simulink model "ModeAdjust"  (R2018b)
settings: Solver=FixedStepDiscrete  StartTime=0.0  StopTime=inf  FixedStep=0.01  RelTol=1e-3
undefined symbols (not defined in the file or in its folder): IfKeSMSbSeatMovBkRclnEnable_Val, IfKeSMSbSeatMovFrwdBkwdEnable_Val, IfKeSMSbSeatMovFtrstEnable_Val, IfKeSMSbSeatMovHdrstFrwdBkwdEnable_Val, IfKeSMSbSeatMovHdUpwdDnwdEnable_Val, IfKeSMSbSeatMovLgrstEnable_Val, IfKeSMSbSeatMovLtwdRtwdEnable_Val, IfVeSMSeStNumConfig, KeSMSbArmscreenMovEnable_Val, KeSMSbSeatMovLgrstExpdEnable_Val, KeSMSuFirstRwStBackPosDelta_Val, KeSMSuFirstRwStBackPosTolr_Val, KeSMSuFirstRwStCushFrntPosDelta_Val, KeSMSuFirstRwStCushFrntPosTolr_Val, KeSMSuFirstRwStCushRePosDelta_Val, KeSMSuFirstRwStCushRePosTolr_Val, KeSMSuFirstRwStFootrestPosDelta_Val, KeSMSuFirstRwStFootrestPosTolr_Val, KeSMSuFirstRwStFwdBkwdPosDelta_Val, KeSMSuFirstRwStFwdBkwdPosTolr_Val, KeSMSuMdMotFinshdTm_Val, KeSMSuMdRetryTm1_Val, KeSMSuModeReqDurgTm_Val, KeSMSuSecRwStArmTochPosDelta_Val, KeSMSuSecRwStArmTochPosTolr_Val, KeSMSuSecRwStBackPosDelta_Val, KeSMSuSecRwStBackPosTolr_Val, KeSMSuSecRwStFtrstUpwdDnwdPosDelta_Val, KeSMSuSecRwStFtrstUpwdDnwdPosTolr_Val, KeSMSuSecRwStFwdBkwdPosDelta_Val, KeSMSuSecRwStFwdBkwdPosTolr_Val, KeSMSuSecRwStHeadrestFwdBkwdPosDelta_Val, KeSMSuSecRwStHeadrestFwdBkwdPosTolr_Val, KeSMSuSecRwStHeadrestUpwdDwnwdPosDelta_Val, KeSMSuSecRwStHeadrestUpwdDwnwdPosTolr_Val, KeSMSuSecRwStLegrestInOutPosDelta_Val, KeSMSuSecRwStLegrestInOutPosTolr_Val, KeSMSuSecRwStLegrestUpwdDwnwdPosDelta_Val, KeSMSuSecRwStLegrestUpwdDwnwdPosTolr_Val, KeSMSuSecRwStLwdRwdPosDelta_Val, KeSMSuSecRwStLwdRwdPosTolr_Val, KeSMSuSecRwStVIPFtrstRefAngle_Val, KeSMSuThirdRwStFwdBkwdPosDelta_Val, KeSMSuThirdRwStFwdBkwdPosTolr_Val, KeSMSuThrdRwCushFoldPosDelta_Val, KeSMSuThrdRwCushFoldPosTolr_Val, KeSMSuThrdRwStBackPosDelta_Val, KeSMSuThrdRwStBackPosTolr_Val, KeSMSw4SLegrstCloseMdSecRwLtStFtrstUpwdDnwdPos_Val, KeSMSw4SLegrstCloseMdSecRwLtStFtrstUpwdDnwdPosMax_Val, KeSMSw4SLegrstCloseMdSecRwLtStFtrstUpwdDnwdPosMin_Val, KeSMSw4SLegrstCloseMdSecRwLtStLgrstOtwdInwdPos_Val, KeSMSw4SLegrstCloseMdSecRwLtStLgrstOtwdInwdPosMax_Val, KeSMSw4SLegrstCloseMdSecRwLtStLgrstOtwdInwdPosMin_Val, KeSMSw4SLegrstCloseMdSecRwLtStLgrstUpwdDnwdPos_Val, KeSMSw4SLegrstCloseMdSecRwLtStLgrstUpwdDnwdPosMax_Val, KeSMSw4SLegrstCloseMdSecRwLtStLgrstUpwdDnwdPosMin_Val, KeSMSw4SLegrstCloseMdSecRwRtStFtrstUpwdDnwdPos_Val, KeSMSw4SLegrstCloseMdSecRwRtStFtrstUpwdDnwdPosMax_Val, KeSMSw4SLegrstCloseMdSecRwRtStFtrstUpwdDnwdPosMin_Val ... (+1138)
libraries: Lib x401
(part 18 of 35)

== system ModeAdjust/ModeAdjustRunnable_sys/ModeAdjust/LgrstOpenL/R2Lt ==
  note: 2L 扶手屏位置
  Mode_Trig : Inport
  SecRwLtStsPoss : Inport  Port=2
  SecRwLtStPossV : Inport  Port=3
  ModeStCalib_2L : Inport  Port=4
  StConfig : Inport  Port=5
  SecRwLtStsPoss4s : Inport  Port=6
  SecRwLtStPossV4s : Inport  Port=7
  StConfig4s : Inport  Port=8
  StepEn_LgrstStep1 : Inport  Port=9
  StepEn_LgrstStep2 : Inport  Port=10
  StepEn_LgrstStep3 : Inport  Port=11
  Bus Creator : BusCreator  Inputs=9  OutDataTypeStr=Bus: SecRwLfSeatPos
  Bus Creator1 : BusCreator  Inputs=3
  Bus Selector : BusSelector  OutputSignals=IfVeSMSuSecRwLtStBkReclnUpwdDnwdPos_Val_read,IfVeSMSuSecRwLtStFrwdBkwdPos_Val_read,IfVeSMSuSecRwLtStHPassStUpwdDnwdPos_Val_read,IfVeSMSuSecRwLtStLgrstUpwdDnwdPos_Val_read,IfVeSMSuSecRwLtStLtwdRtwdPos_Val_read,IfVeSMSuSecRwLtStArmScrnPos_Val_read
  Bus Selector1 : BusSelector  OutputSignals=IfVeSMSuSecRwLtStBkReclnUpwdDnwdPosV_Val_read,IfVeSMSuSecRwLtStFrwdBkwdPosV_Val_read,IfVeSMSuSecRwLtStHPassStUpwdDnwdPosV_Val_read,IfVeSMSuSecRwLtStLgrstUpwdDnwdPosV_Val_read,IfVeSMSuSecRwLtStLtwdRtwdPosV_Val_read,IfVeSMSuSecRwLtStArmScrnPosV_Val_read
  Bus Selector2 : BusSelector  OutputSignals=BkReclnUpwdDnwdPos,BkReclnUpwdDnwdPosMax,BkReclnUpwdDnwdPosMin,HdrstUpwdPos,HdrstUpwdPosMax,HdrstUpwdPosMin,LgrstUpwdPos,LgrstUpwdPosMax,LgrstUpwdPosMin,LgrstOtwdInwdPos,LgrstOtwdInwdPosMax,LgrstOtwdInwdPosMin,FtrstUpwdDnwdPos,FtrstUpwdDnwdPosMax,FtrstUpwdDnwdPosMin,HdrstFrwdBkwdnwdPos,HdrstFrwdBkwdnwdPosMax,HdrstFrwdBkwdnwdPosMin
  Bus Selector3 : BusSelector  OutputSignals=LgrstOpenLSecRwLtSt
  Bus Selector4 : BusSelector  OutputSignals=BkReclnUpwdDnwdMovConfig,ArmTouchMovConfig,FrwdBkwdMovConfig,LgrstUpwdMovConfig,LtwdRtwdMovConfig
  Bus Selector5 : BusSelector  OutputSignals=IfVeSMSuSecRwLtStLgrstOtwdInwdPos_Val_read,IfVeSMSuRrLtStFtUpwdDnwdPos_Val_read,IfVeSMSuSecRwLtStHdrstFrwdBkwdPos_Val_read
  Bus Selector6 : BusSelector  OutputSignals=IfVeSMSuSecRwLtStLgrstOtwdInwdPosV_Val_read,IfVeSMSuRrLtStFtUpwdDnwdPosV_Val_read,IfVeSMSuSecRwLtStHdrstFrwdBkwdPosV_Val_read
  Bus Selector7 : BusSelector  OutputSignals=LgrstExpdMovConfig,FtrstMovConfig,HdrstUpwdDnwdMovConfig,HdrstFrwdBkwdMovConfig
  Logical Operator10 : Logic  AllPortsSameDT=off  OutDataTypeStr=boolean
  Logical Operator4 : Logic  Operator=OR  AllPortsSameDT=off  OutDataTypeStr=boolean
  Logical Operator5 : Logic  Operator=OR  AllPortsSameDT=off  OutDataTypeStr=boolean
  Logical Operator6 : Logic  Operator=OR  AllPortsSameDT=off  OutDataTypeStr=boolean
  PA_KeSMSuMdMotFinshdTm_Val : Constant  Value=KeSMSuMdMotFinshdTm_Val
  PA_KeSMSuMdRetryTm1_Val : Constant  Value=KeSMSuMdRetryTm1_Val
  PA_KeSMSuModeReqDurgTm_Val : Constant  Value=KeSMSuModeReqDurgTm_Val
  PA_KeSMSuSecRwStBackPosDelta_Val : Constant  Value=KeSMSuSecRwStBackPosDelta_Val
  PA_KeSMSuSecRwStFtrstUpwdDnwdPosDelta_Val : Constant  Value=KeSMSuSecRwStFtrstUpwdDnwdPosDelta_Val
  PA_KeSMSuSecRwStHeadrestFwdBkwdPosDelta_Val : Constant  Value=KeSMSuSecRwStHeadrestFwdBkwdPosDelta_Val
  PA_KeSMSuSecRwStHeadrestUpwdDwnwdPosDelta_Val : Constant  Value=KeSMSuSecRwStHeadrestUpwdDwnwdPosDelta_Val
  PA_KeSMSuSecRwStLegrestInOutPosDelta_Val : Constant  Value=KeSMSuSecRwStLegrestInOutPosDelta_Val
  PA_KeSMSuSecRwStLegrestUpwdDwnwdPosDelta_Val : Constant  Value=KeSMSuSecRwStLegrestUpwdDwnwdPosDelta_Val
  PA_KeSMSwDltTrgtPos_Val{1,3,5..8,12..13,16,18..20} (12 alike) : Constant  Value=KeSMSwPosInvalidVal_Val
  PA_KeSMSwDltTrgtPos_Val{9..11,14..15,22} (6 alike) : Constant  Value=0  OutDataTypeStr=boolean
  PA_KeSMSwDltTrgtPos_Val4 : Constant  OutDataTypeStr=boolean
  SecRwLtStFtUpwd_Lt_Step2 : Lib/CommonUsed  SystemSampleTime=-1
  SecRwLtStLgrstOtwd_Lt_Step1 : Lib/CommonUsed  SystemSampleTime=-1
  SecRwLtStLgrstUpwd_Lt_Step3 : Lib/CommonUsed  SystemSampleTime=-1
  Unit Delay : UnitDelay  SampleTime=-1
  Unit Delay1 : UnitDelay  SampleTime=-1
  Unit Delay2 : UnitDelay  SampleTime=-1
  R2Lt_TrgtPoss : Outport  VectorParamsAs1DForOutWhenUnconnected=on
  IfVeSMSuSecRwLtStRclCmdSrv_Val_writeRaw : Outport  Port=2
  lgrstStep1_ini : Outport  Port=3  VectorParamsAs1DForOutWhenUnconnected=on
  lgrstStep2_ini : Outport  Port=4  VectorParamsAs1DForOutWhenUnconnected=on
  lgrstStep3_ini : Outport  Port=5  VectorParamsAs1DForOutWhenUnconnected=on
  lgrstStep1_done : Outport  Port=6  VectorParamsAs1DForOutWhenUnconnected=on
  lgrstStep2_done : Outport  Port=7  VectorParamsAs1DForOutWhenUnconnected=on
  lgrstStep3_done : Outport  Port=8  VectorParamsAs1DForOutWhenUnconnected=on
  R2Lt_TrgtPoss_2 : Outport  Port=9  VectorParamsAs1DForOutWhenUnconnected=on
  wires:
  PA_KeSMSuSecRwStHeadrestFwdBkwdPosDelta_Val/1 -> [KeSMSuSecRwStHeadrestFwdBkwdPosDelta_Val]
  Bus Selector2/18 -> [K_HdrstFrwdBkwdnwdPosMin]  "<HdrstFrwdBkwdnwdPosMin>"
  Bus Selector2/17 -> [K_HdrstFrwdBkwdnwdPosMax]  "<HdrstFrwdBkwdnwdPosMax>"
  Bus Selector2/16 -> [K_HdrstFrwdBkwdnwdPos]  "<HdrstFrwdBkwdnwdPos>"
  Bus Selector6/3 -> [SecRwLtStHdrstFrwdBkwdPosV]  "<IfVeSMSuSecRwLtStHdrstFrwdBkwdPosV_Val_read>"
  Bus Selector5/3 -> [SecRwLtStHdrstFrwdBkwdPos]  "<IfVeSMSuSecRwLtStHdrstFrwdBkwdPos_Val_read>"
  Bus Selector7/4 -> [HdrstFrwdBkwdMovConfig]  "<HdrstFrwdBkwdMovConfig>"
  PA_KeSMSwDltTrgtPos_Val6/1 -> Bus Creator1/3  "SecRwLtStHdrstFrwdBkwdTrgtPos"
  PA_KeSMSuMdRetryTm1_Val/1 -> [CntLow]
  [CntLow] -> SecRwLtStLgrstUpwd_Lt_Step3/15
  [CntLow] -> SecRwLtStLgrstOtwd_Lt_Step1/15
  [CntLow] -> SecRwLtStFtUpwd_Lt_Step2/15
  PA_KeSMSwDltTrgtPos_Val4/1 -> IfVeSMSuSecRwLtStRclCmdSrv_Val_writeRaw/1
  SecRwLtStLgrstUpwd_Lt_Step3/1 -> [lgrstStep1_ini]
  Mode_Trig/1 -> [Trig]
  Bus Selector1/3 -> [SecRwLtStHPassStUpwdDnwdPosV]  "<IfVeSMSuSecRwLtStHPassStUpwdDnwdPosV_Val_read>"
  Bus Selector/5 -> [SecRwLtStLtwdRtwdPos]  "<IfVeSMSuSecRwLtStLtwdRtwdPos_Val_read>"
  SecRwLtStsPoss/1 -> Bus Selector/1
  Bus Selector1/4 -> [SecRwLtStLgrstUpwdDnwdPosV]  "<IfVeSMSuSecRwLtStLgrstUpwdDnwdPosV_Val_read>"
  SecRwLtStPossV/1 -> Bus Selector1/1
  Bus Selector/3 -> [SecRwLtStHPassStUpwdDnwdPos]  "<IfVeSMSuSecRwLtStHPassStUpwdDnwdPos_Val_read>"
  Bus Selector1/5 -> [SecRwLtStLtwdRtwdPosV]  "<IfVeSMSuSecRwLtStLtwdRtwdPosV_Val_read>"
  Bus Selector/4 -> [SecRwLtStLgrstUpwdDnwdPos]  "<IfVeSMSuSecRwLtStLgrstUpwdDnwdPos_Val_read>"
  Bus Selector/2 -> [SecRwLtStFrwdBkwdPos]  "<IfVeSMSuSecRwLtStFrwdBkwdPos_Val_read>"
  Bus Selector1/1 -> [SecRwLtStBkReclnUpwdDnwdPosV]  "<IfVeSMSuSecRwLtStBkReclnUpwdDnwdPosV_Val_read>"
  Bus Selector1/2 -> [SecRwLtStFrwdBkwdPosV]  "<IfVeSMSuSecRwLtStFrwdBkwdPosV_Val_read>"
  Bus Selector/1 -> [SecRwLtStBkReclnUpwdDnwdPos]  "<IfVeSMSuSecRwLtStBkReclnUpwdDnwdPos_Val_read>"
  [Trig] -> SecRwLtStLgrstUpwd_Lt_Step3/1
  [StepEn_LgrstStep1] -> SecRwLtStLgrstUpwd_Lt_Step3/2
  [K_LgrstUpwdPosMin] -> SecRwLtStLgrstUpwd_Lt_Step3/4
  [K_LgrstUpwdPosMax] -> SecRwLtStLgrstUpwd_Lt_Step3/5
  [K_LgrstUpwdPos] -> SecRwLtStLgrstUpwd_Lt_Step3/6
  [SecRwLtStLgrstUpwdDnwdPos] -> SecRwLtStLgrstUpwd_Lt_Step3/3
  [KeSMSuSecRwStLegrestUpwdDwnwdPosDelta_Val] -> SecRwLtStLgrstUpwd_Lt_Step3/7
  [SecRwLtStLgrstUpwdDnwdPosV] -> SecRwLtStLgrstUpwd_Lt_Step3/8
  PA_KeSMSwDltTrgtPos_Val10/1 -> SecRwLtStLgrstUpwd_Lt_Step3/9
  PA_KeSMSwDltTrgtPos_Val12/1 -> SecRwLtStLgrstUpwd_Lt_Step3/10
  [Tick] -> SecRwLtStLgrstUpwd_Lt_Step3/11
  SecRwLtStLgrstUpwd_Lt_Step3/2 -> [lgrst_ArrivedTarPos]
  SecRwLtStLgrstUpwd_Lt_Step3/3 -> [R2Lt_LgrstUpwd_TarPos]
  SecRwLtStLgrstUpwd_Lt_Step3/4 -> [lgrstStep1_done]
  PA_KeSMSwDltTrgtPos_Val3/1 -> Bus Creator/6  "SecRwLtStHdrstUpwdDnwdTrgtPos"
  Bus Creator/1 -> R2Lt_TrgtPoss/1
  [R2Lt_LgrstUpwd_TarPos] -> Bus Creator/7  "SecRwLtStLgrstUpwdDnwdTrgtPos"
  PA_KeSMSwDltTrgtPos_Val19/1 -> Bus Creator/3  "SecRwLtStCshnFrntUpwdDnwdTrgtPos"
  PA_KeSMSwDltTrgtPos_Val1/1 -> Bus Creator/8  "SecRwLtStLtwdRtwdTrgtPos"
  PA_KeSMSwDltTrgtPos_Val18/1 -> Bus Creator/2  "SecRwLtStBlstOtwdInwdTrgtPos"
  PA_KeSMSwDltTrgtPos_Val5/1 -> Bus Creator/1  "SecRwLtStBkReclnUpwdDnwdTrgtPos"
  PA_KeSMSwDltTrgtPos_Val8/1 -> Bus Creator/5  "SecRwLtStFrwdBkwdTrgtPos"
  PA_KeSMSwDltTrgtPos_Val20/1 -> Bus Creator/4  "SecRwLtStCshnRrUpwdDnwdTrgtPos"
  PA_KeSMSuModeReqDurgTm_Val/1 -> [Tick]
  PA_KeSMSwDltTrgtPos_Val7/1 -> Bus Creator/9  "SecRwLtStArmScrnTrgtPos"
  PA_KeSMSuSecRwStBackPosDelta_Val/1 -> [KeSMSuSecRwStBackPosDelta_Val]
  PA_KeSMSuSecRwStLegrestUpwdDwnwdPosDelta_Val/1 -> [KeSMSuSecRwStLegrestUpwdDwnwdPosDelta_Val]
  PA_KeSMSuMdMotFinshdTm_Val/1 -> [KeSMSuMdMotFinshdTm_Val]
  [KeSMSuMdMotFinshdTm_Val] -> SecRwLtStLgrstUpwd_Lt_Step3/12
  Bus Selector/6 -> [R2LtStArmScrnPos]  "<IfVeSMSuSecRwLtStArmScrnPos_Val_read>"
  Bus Selector1/6 -> [R2LtStArmScrnPosV]  "<IfVeSMSuSecRwLtStArmScrnPosV_Val_read>"
  Bus Selector2/9 -> [K_LgrstUpwdPosMin]  "<LgrstUpwdPosMin>"
  Bus Selector2/6 -> [K_HdrstUpwdPosMin]  "<HdrstUpwdPosMin>"
  Bus Selector2/7 -> [K_LgrstUpwdPos]  "<LgrstUpwdPos>"
  Bus Selector2/5 -> [K_HdrstUpwdPosMax]  "<HdrstUpwdPosMax>"
  Bus Selector2/8 -> [K_LgrstUpwdPosMax]  "<LgrstUpwdPosMax>"
  Bus Selector2/4 -> [K_HdrstUpwdPos]  "<HdrstUpwdPos>"
  Bus Selector2/1 -> [K_BkReclnUpwdDnwdPos]  "<BkReclnUpwdDnwdPos>"
  Bus Selector2/2 -> [K_BkReclnUpwdDnwdPosMax]  "<BkReclnUpwdDnwdPosMax>"
  Bus Selector3/1 -> Bus Selector2/1  "<LgrstOpenLSecRwLtSt>"
  Bus Selector2/3 -> [K_BkReclnUpwdDnwdPosMin]  "<BkReclnUpwdDnwdPosMin>"
  ModeStCalib_2L/1 -> Bus Selector3/1
  StConfig/1 -> Bus Selector4/1
  Bus Selector4/3 -> [FrwdBkwdMovConfig]  "<FrwdBkwdMovConfig>"
  Bus Selector4/5 -> [LtwdRtwdMovConfig]  "<LtwdRtwdMovConfig>"
  Bus Selector4/4 -> [LgrstUpwdMovConfig]  "<LgrstUpwdMovConfig>"
  Bus Selector4/2 -> [ArmTouchMovConfig]  "<ArmTouchMovConfig>"
  Bus Selector4/1 -> [BkReclnUpwdDnwdMovConfig]  "<BkReclnUpwdDnwdMovConfig>"
  PA_KeSMSwDltTrgtPos_Val9/1 -> SecRwLtStLgrstUpwd_Lt_Step3/13
  [LgrstUpwdMovConfig] -> SecRwLtStLgrstUpwd_Lt_Step3/14
  Bus Selector2/10 -> [K_LgrstOtwdInwdPos]  "<LgrstOtwdInwdPos>"
  Bus Selector2/11 -> [K_LgrstOtwdInwdPosMax]  "<LgrstOtwdInwdPosMax>"
  Bus Selector2/12 -> [K_LgrstOtwdInwdPosMin]  "<LgrstOtwdInwdPosMin>"
  Bus Selector2/15 -> [K_FtrstUpwdPosMin]  "<FtrstUpwdDnwdPosMin>"
  Bus Selector2/14 -> [K_FtrstUpwdPosMax]  "<FtrstUpwdDnwdPosMax>"
  Bus Selector2/13 -> [K_FtrstUpwdPos]  "<FtrstUpwdDnwdPos>"
  PA_KeSMSuSecRwStFtrstUpwdDnwdPosDelta_Val/1 -> [KeSMSuSecRwStFtrstUpwdDnwdPosDelta_Val]
  PA_KeSMSuSecRwStHeadrestUpwdDwnwdPosDelta_Val/1 -> [KeSMSuSecRwStHeadrestUpwdDwnwdPosDelta_Val]
  PA_KeSMSuSecRwStLegrestInOutPosDelta_Val/1 -> [KeSMSuSecRwStLegrestInOutPosDelta_Val]
  SecRwLtStsPoss4s/1 -> Bus Selector5/1
  SecRwLtStPossV4s/1 -> Bus Selector6/1
  Bus Selector5/1 -> [SecRwLtStLgrstOtwdInwdPos]  "<IfVeSMSuSecRwLtStLgrstOtwdInwdPos_Val_read>"
  Bus Selector5/2 -> [RrLtStFtUpwdDnwdPos]  "<IfVeSMSuRrLtStFtUpwdDnwdPos_Val_read>"
  Bus Selector6/1 -> [SecRwLtStLgrstOtwdInwdPosV]  "<IfVeSMSuSecRwLtStLgrstOtwdInwdPosV_Val_read>"
  Bus Selector6/2 -> [RrLtStFtUpwdDnwdPosV]  "<IfVeSMSuRrLtStFtUpwdDnwdPosV_Val_read>"
  [LgrstExpdMovConfig] -> SecRwLtStLgrstOtwd_Lt_Step1/14
  PA_KeSMSwDltTrgtPos_Val15/1 -> SecRwLtStLgrstOtwd_Lt_Step1/13
  [KeSMSuMdMotFinshdTm_Val] -> SecRwLtStLgrstOtwd_Lt_Step1/12
  SecRwLtStLgrstOtwd_Lt_Step1/4 -> [LgrstStep3_1_done]
  SecRwLtStLgrstOtwd_Lt_Step1/3 -> [R2Lt_LgrstOtwd_TarPos]
  SecRwLtStLgrstOtwd_Lt_Step1/2 -> [LgOt_ArrivedTarPos]
  [Tick] -> SecRwLtStLgrstOtwd_Lt_Step1/11
  PA_KeSMSwDltTrgtPos_Val13/1 -> SecRwLtStLgrstOtwd_Lt_Step1/10
  PA_KeSMSwDltTrgtPos_Val14/1 -> SecRwLtStLgrstOtwd_Lt_Step1/9
  [SecRwLtStLgrstOtwdInwdPosV] -> SecRwLtStLgrstOtwd_Lt_Step1/8
  [KeSMSuSecRwStLegrestInOutPosDelta_Val] -> SecRwLtStLgrstOtwd_Lt_Step1/7
  [SecRwLtStLgrstOtwdInwdPos] -> SecRwLtStLgrstOtwd_Lt_Step1/3
  [K_LgrstOtwdInwdPos] -> SecRwLtStLgrstOtwd_Lt_Step1/6
  [K_LgrstOtwdInwdPosMax] -> SecRwLtStLgrstOtwd_Lt_Step1/5
  [K_LgrstOtwdInwdPosMin] -> SecRwLtStLgrstOtwd_Lt_Step1/4
  [StepEn_LgrstStep3] -> SecRwLtStLgrstOtwd_Lt_Step1/2
  [Trig] -> SecRwLtStLgrstOtwd_Lt_Step1/1
  SecRwLtStLgrstOtwd_Lt_Step1/1 -> [LgrstStep3_1_ini]
  SecRwLtStFtUpwd_Lt_Step2/1 -> [LgrstStep2_1_ini]
  [Trig] -> SecRwLtStFtUpwd_Lt_Step2/1
  [StepEn_LgrstStep2] -> SecRwLtStFtUpwd_Lt_Step2/2
  [K_FtrstUpwdPosMin] -> SecRwLtStFtUpwd_Lt_Step2/4
  [K_FtrstUpwdPosMax] -> SecRwLtStFtUpwd_Lt_Step2/5
  [K_FtrstUpwdPos] -> SecRwLtStFtUpwd_Lt_Step2/6
  [RrLtStFtUpwdDnwdPos] -> SecRwLtStFtUpwd_Lt_Step2/3
  [KeSMSuSecRwStFtrstUpwdDnwdPosDelta_Val] -> SecRwLtStFtUpwd_Lt_Step2/7
  [RrLtStFtUpwdDnwdPosV] -> SecRwLtStFtUpwd_Lt_Step2/8
  PA_KeSMSwDltTrgtPos_Val11/1 -> SecRwLtStFtUpwd_Lt_Step2/9
  PA_KeSMSwDltTrgtPos_Val16/1 -> SecRwLtStFtUpwd_Lt_Step2/10
  [Tick] -> SecRwLtStFtUpwd_Lt_Step2/11
  SecRwLtStFtUpwd_Lt_Step2/2 -> [Ft_ArrivedTarPos]
  SecRwLtStFtUpwd_Lt_Step2/3 -> [R2Lt_FtUpwd_TarPos]
  SecRwLtStFtUpwd_Lt_Step2/4 -> [LgrstStep2_1_done]
  [KeSMSuMdMotFinshdTm_Val] -> SecRwLtStFtUpwd_Lt_Step2/12
  PA_KeSMSwDltTrgtPos_Val22/1 -> SecRwLtStFtUpwd_Lt_Step2/13
  [FtrstMovConfig] -> SecRwLtStFtUpwd_Lt_Step2/14
  StConfig4s/1 -> Bus Selector7/1
  Bus Selector7/1 -> [LgrstExpdMovConfig]  "<LgrstExpdMovConfig>"
  Bus Selector7/2 -> [FtrstMovConfig]  "<FtrstMovConfig>"
  Bus Selector7/3 -> [HdrstMovConfig]  "<HdrstUpwdDnwdMovConfig>"
  [lgrstStep1_ini] -> lgrstStep1_ini/1
  [LgrstStep2_1_ini] -> lgrstStep2_ini/1
  [LgrstStep3_1_ini] -> lgrstStep3_ini/1
  StepEn_LgrstStep1/1 -> [StepEn_LgrstStep1]
  StepEn_LgrstStep2/1 -> [StepEn_LgrstStep2]
  StepEn_LgrstStep3/1 -> [StepEn_LgrstStep3]
  [LgrstStep2_1_done] -> Unit Delay1/1
  Logical Operator4/1 -> lgrstStep1_done/1
  [lgrstStep1_done] -> Unit Delay/1
  [lgrstStep1_ini] -> Logical Operator4/1
  Unit Delay/1 -> Logical Operator4/2
  Logical Operator5/1 -> [lgrst_Step2done], lgrstStep2_done/1
  Unit Delay1/1 -> Logical Operator5/2
  Logical Operator6/1 -> lgrstStep3_done/1
  Unit Delay2/1 -> Logical Operator6/2
  [LgrstStep3_1_done] -> Logical Operator10/2
  Logical Operator10/1 -> Unit Delay2/1
  [lgrst_Step2done] -> Logical Operator10/1
  [LgrstStep2_1_ini] -> Logical Operator5/1
  [LgrstStep3_1_ini] -> Logical Operator6/1
  Bus Creator1/1 -> R2Lt_TrgtPoss_2/1
  [R2Lt_FtUpwd_TarPos] -> Bus Creator1/1  "RrLtStFtUpwdDnwdTrgtPos"
  [R2Lt_LgrstOtwd_TarPos] -> Bus Creator1/2  "SecRwLtStLgrstOtwdInwdTrgtPos"

== system ModeAdjust/ModeAdjustRunnable_sys/ModeAdjust/LgrstOpenR/R2Lt ==
  note: 2L 扶手屏位置
  Mode_Trig : Inport
  SecRwLtStsPoss : Inport  Port=2
  SecRwLtStPossV : Inport  Port=3
  ModeStCalib_2L : Inport  Port=4
  StConfig : Inport  Port=5
  SecRwLtStsPoss4s : Inport  Port=6
  SecRwLtStPossV4s : Inport  Port=7
  StConfig4s : Inport  Port=8
  StepEn_LgrstStep1 : Inport  Port=9
  StepEn_LgrstStep2 : Inport  Port=10
  StepEn_LgrstStep3 : Inport  Port=11
  Bus Creator : BusCreator  Inputs=9  OutDataTypeStr=Bus: SecRwRtSeatPos
  Bus Creator1 : BusCreator  Inputs=3
  Bus Selector : BusSelector  OutputSignals=IfVeSMSuSecRwRtStBkReclnUpwdDnwdPos_Val_read,IfVeSMSuSecRwRtStFrwdBkwdPos_Val_read,IfVeSMSuSecRwRtStHPassStUpwdDnwdPos_Val_read,IfVeSMSuSecRwRtStLgrstUpwdDnwdPos_Val_read,IfVeSMSuSecRwRtStLtwdRtwdPos_Val_read,SecRwRtStArmScrnPos_Val_read
  Bus Selector1 : BusSelector  OutputSignals=IfVeSMSuSecRwRtStBkReclnUpwdDnwdPosV_Val_read,IfVeSMSuSecRwRtStFrwdBkwdPosV_Val_read,IfVeSMSuSecRwRtStHPassStUpwdDnwdPosV_Val_read,IfVeSMSuSecRwRtStLgrstUpwdDnwdPosV_Val_read,IfVeSMSuSecRwRtStLtwdRtwdPosV_Val_read,SecRwRtStArmScrnPosV_Val_read
  Bus Selector2 : BusSelector  OutputSignals=BkReclnUpwdDnwdPos,BkReclnUpwdDnwdPosMax,BkReclnUpwdDnwdPosMin,HdrstUpwdPos,HdrstUpwdPosMax,HdrstUpwdPosMin,LgrstUpwdPos,LgrstUpwdPosMax,LgrstUpwdPosMin,LgrstOtwdInwdPos,LgrstOtwdInwdPosMax,LgrstOtwdInwdPosMin,FtrstUpwdDnwdPos,FtrstUpwdDnwdPosMax,FtrstUpwdDnwdPosMin,HdrstFrwdBkwdnwdPos,HdrstFrwdBkwdnwdPosMax,HdrstFrwdBkwdnwdPosMin
  Bus Selector3 : BusSelector  OutputSignals=LgrstOpenRSecRwRtSt
  Bus Selector4 : BusSelector  OutputSignals=BkReclnUpwdDnwdMovConfig,ArmTouchMovConfig,FrwdBkwdMovConfig,LgrstUpwdMovConfig,LtwdRtwdMovConfig
  Bus Selector5 : BusSelector  OutputSignals=IfVeSMSuSecRwRtStLgrstOtwdInwdPos_Val_read,IfVeSMSuRrRtStFtUpwdDnwdPos_Val_read,IfVeSMSuSecRwRtStHdrstFrwdBkwdPos_Val_read
  Bus Selector6 : BusSelector  OutputSignals=IfVeSMSuSecRwRtStLgrstOtwdInwdPosV_Val_read,IfVeSMSuRrRtStFtUpwdDnwdPosV_Val_read,IfVeSMSuSecRwRtStHdrstFrwdBkwdPosV_Val_read
  Bus Selector7 : BusSelector  OutputSignals=LgrstExpdMovConfig,FtrstMovConfig,HdrstUpwdDnwdMovConfig,HdrstFrwdBkwdMovConfig
  Logical Operator10 : Logic  AllPortsSameDT=off  OutDataTypeStr=boolean
  Logical Operator4 : Logic  Operator=OR  AllPortsSameDT=off  OutDataTypeStr=boolean
  Logical Operator5 : Logic  Operator=OR  AllPortsSameDT=off  OutDataTypeStr=boolean
  Logical Operator6 : Logic  Operator=OR  AllPortsSameDT=off  OutDataTypeStr=boolean
  PA_KeSMSuMdMotFinshdTm_Val : Constant  Value=KeSMSuMdMotFinshdTm_Val
  PA_KeSMSuMdRetryTm1_Val : Constant  Value=KeSMSuMdRetryTm1_Val
  PA_KeSMSuModeReqDurgTm_Val : Constant  Value=KeSMSuModeReqDurgTm_Val
  PA_KeSMSuSecRwStBackPosDelta_Val : Constant  Value=KeSMSuSecRwStBackPosDelta_Val
  PA_KeSMSuSecRwStFtrstUpwdDnwdPosDelta_Val : Constant  Value=KeSMSuSecRwStFtrstUpwdDnwdPosDelta_Val
  PA_KeSMSuSecRwStHeadrestFwdBkwdPosDelta_Val : Constant  Value=KeSMSuSecRwStHeadrestFwdBkwdPosDelta_Val
  PA_KeSMSuSecRwStHeadrestUpwdDwnwdPosDelta_Val : Constant  Value=KeSMSuSecRwStHeadrestUpwdDwnwdPosDelta_Val
  PA_KeSMSuSecRwStLegrestInOutPosDelta_Val : Constant  Value=KeSMSuSecRwStLegrestInOutPosDelta_Val
  PA_KeSMSuSecRwStLegrestUpwdDwnwdPosDelta_Val : Constant  Value=KeSMSuSecRwStLegrestUpwdDwnwdPosDelta_Val
  PA_KeSMSwDltTrgtPos_Val{1,3,5..8,12..13,16,18..20} (12 alike) : Constant  Value=KeSMSwPosInvalidVal_Val
  PA_KeSMSwDltTrgtPos_Val{9..11,14..15,22} (6 alike) : Constant  Value=0  OutDataTypeStr=boolean
  PA_KeSMSwDltTrgtPos_Val4 : Constant  OutDataTypeStr=boolean
  SecRwLtStFtUpwd_Lt_Step2 : Lib/CommonUsed  SystemSampleTime=-1
  SecRwLtStLgrstOtwd_Lt_Step1 : Lib/CommonUsed  SystemSampleTime=-1
  SecRwLtStLgrstUpwd_Lt_Step3 : Lib/CommonUsed  SystemSampleTime=-1
  Unit Delay : UnitDelay  SampleTime=-1
  Unit Delay1 : UnitDelay  SampleTime=-1
  Unit Delay2 : UnitDelay  SampleTime=-1
  R2Rt_TrgtPoss : Outport  VectorParamsAs1DForOutWhenUnconnected=on
  IfVeSMSuSecRwLtStRclCmdSrv_Val_writeRaw : Outport  Port=2
  lgrstStep1_ini : Outport  Port=3  VectorParamsAs1DForOutWhenUnconnected=on
  lgrstStep2_ini : Outport  Port=4  VectorParamsAs1DForOutWhenUnconnected=on
  lgrstStep3_ini : Outport  Port=5  VectorParamsAs1DForOutWhenUnconnected=on
  lgrstStep1_done : Outport  Port=6  VectorParamsAs1DForOutWhenUnconnected=on
  lgrstStep2_done : Outport  Port=7  VectorParamsAs1DForOutWhenUnconnected=on
  lgrstStep3_done : Outport  Port=8  VectorParamsAs1DForOutWhenUnconnected=on
  R2Rt_TrgtPoss_2 : Outport  Port=9  VectorParamsAs1DForOutWhenUnconnected=on
  wires:
  [R2Lt_LgrstOtwd_TarPos] -> Bus Creator1/2  "SecRwRtStLgrstOtwdInwdTrgtPos"
  [R2Lt_FtUpwd_TarPos] -> Bus Creator1/1  "RrRtStFtUpwdDnwdTrgtPos"
  Bus Creator1/1 -> R2Rt_TrgtPoss_2/1
  [LgrstStep3_1_ini] -> Logical Operator6/1
  [LgrstStep2_1_ini] -> Logical Operator5/1
  [lgrst_Step2done] -> Logical Operator10/1
  Logical Operator10/1 -> Unit Delay2/1
  [LgrstStep3_1_done] -> Logical Operator10/2
  Unit Delay2/1 -> Logical Operator6/2
  Logical Operator6/1 -> lgrstStep3_done/1
  Unit Delay1/1 -> Logical Operator5/2
  Logical Operator5/1 -> lgrstStep2_done/1, [lgrst_Step2done]
  Unit Delay/1 -> Logical Operator4/2
  [lgrstStep1_ini] -> Logical Operator4/1
  [lgrstStep1_done] -> Unit Delay/1
  Logical Operator4/1 -> lgrstStep1_done/1
  [LgrstStep2_1_done] -> Unit Delay1/1
  StepEn_LgrstStep3/1 -> [StepEn_LgrstStep3]
  StepEn_LgrstStep2/1 -> [StepEn_LgrstStep2]
  StepEn_LgrstStep1/1 -> [StepEn_LgrstStep1]
  [LgrstStep3_1_ini] -> lgrstStep3_ini/1
  [LgrstStep2_1_ini] -> lgrstStep2_ini/1
  [lgrstStep1_ini] -> lgrstStep1_ini/1
  Bus Selector7/3 -> [HdrstMovConfig]  "<HdrstUpwdDnwdMovConfig>"
  Bus Selector7/2 -> [FtrstMovConfig]  "<FtrstMovConfig>"
  Bus Selector7/1 -> [LgrstExpdMovConfig]  "<LgrstExpdMovConfig>"
  StConfig4s/1 -> Bus Selector7/1
  [FtrstMovConfig] -> SecRwLtStFtUpwd_Lt_Step2/14
  PA_KeSMSwDltTrgtPos_Val22/1 -> SecRwLtStFtUpwd_Lt_Step2/13
  [KeSMSuMdMotFinshdTm_Val] -> SecRwLtStFtUpwd_Lt_Step2/12
  SecRwLtStFtUpwd_Lt_Step2/4 -> [LgrstStep2_1_done]
  SecRwLtStFtUpwd_Lt_Step2/3 -> [R2Lt_FtUpwd_TarPos]
  SecRwLtStFtUpwd_Lt_Step2/2 -> [Ft_ArrivedTarPos]
  [Tick] -> SecRwLtStFtUpwd_Lt_Step2/11
  PA_KeSMSwDltTrgtPos_Val16/1 -> SecRwLtStFtUpwd_Lt_Step2/10
  PA_KeSMSwDltTrgtPos_Val11/1 -> SecRwLtStFtUpwd_Lt_Step2/9
  [RrLtStFtUpwdDnwdPosV] -> SecRwLtStFtUpwd_Lt_Step2/8
  [KeSMSuSecRwStFtrstUpwdDnwdPosDelta_Val] -> SecRwLtStFtUpwd_Lt_Step2/7
  [RrLtStFtUpwdDnwdPos] -> SecRwLtStFtUpwd_Lt_Step2/3
  [K_FtrstUpwdPos] -> SecRwLtStFtUpwd_Lt_Step2/6
  [K_FtrstUpwdPosMax] -> SecRwLtStFtUpwd_Lt_Step2/5
  [K_FtrstUpwdPosMin] -> SecRwLtStFtUpwd_Lt_Step2/4
  [StepEn_LgrstStep2] -> SecRwLtStFtUpwd_Lt_Step2/2
  [Trig] -> SecRwLtStFtUpwd_Lt_Step2/1
  SecRwLtStFtUpwd_Lt_Step2/1 -> [LgrstStep2_1_ini]
  SecRwLtStLgrstOtwd_Lt_Step1/1 -> [LgrstStep3_1_ini]
  [Trig] -> SecRwLtStLgrstOtwd_Lt_Step1/1
  [StepEn_LgrstStep3] -> SecRwLtStLgrstOtwd_Lt_Step1/2
  [K_LgrstOtwdInwdPosMin] -> SecRwLtStLgrstOtwd_Lt_Step1/4
  [K_LgrstOtwdInwdPosMax] -> SecRwLtStLgrstOtwd_Lt_Step1/5
  [K_LgrstOtwdInwdPos] -> SecRwLtStLgrstOtwd_Lt_Step1/6
  [SecRwLtStLgrstOtwdInwdPos] -> SecRwLtStLgrstOtwd_Lt_Step1/3
  [KeSMSuSecRwStLegrestInOutPosDelta_Val] -> SecRwLtStLgrstOtwd_Lt_Step1/7
  [SecRwLtStLgrstOtwdInwdPosV] -> SecRwLtStLgrstOtwd_Lt_Step1/8
  PA_KeSMSwDltTrgtPos_Val14/1 -> SecRwLtStLgrstOtwd_Lt_Step1/9
  PA_KeSMSwDltTrgtPos_Val13/1 -> SecRwLtStLgrstOtwd_Lt_Step1/10
  [Tick] -> SecRwLtStLgrstOtwd_Lt_Step1/11
  SecRwLtStLgrstOtwd_Lt_Step1/2 -> [LgOt_ArrivedTarPos]
  SecRwLtStLgrstOtwd_Lt_Step1/3 -> [R2Lt_LgrstOtwd_TarPos]
  SecRwLtStLgrstOtwd_Lt_Step1/4 -> [LgrstStep3_1_done]
  [KeSMSuMdMotFinshdTm_Val] -> SecRwLtStLgrstOtwd_Lt_Step1/12
  PA_KeSMSwDltTrgtPos_Val15/1 -> SecRwLtStLgrstOtwd_Lt_Step1/13
  [LgrstExpdMovConfig] -> SecRwLtStLgrstOtwd_Lt_Step1/14
  Bus Selector6/2 -> [RrLtStFtUpwdDnwdPosV]  "<IfVeSMSuRrRtStFtUpwdDnwdPosV_Val_read>"
  Bus Selector6/1 -> [SecRwLtStLgrstOtwdInwdPosV]  "<IfVeSMSuSecRwRtStLgrstOtwdInwdPosV_Val_read>"
  Bus Selector5/2 -> [RrLtStFtUpwdDnwdPos]  "<IfVeSMSuRrRtStFtUpwdDnwdPos_Val_read>"
  Bus Selector5/1 -> [SecRwLtStLgrstOtwdInwdPos]  "<IfVeSMSuSecRwRtStLgrstOtwdInwdPos_Val_read>"
  SecRwLtStPossV4s/1 -> Bus Selector6/1
  SecRwLtStsPoss4s/1 -> Bus Selector5/1
  PA_KeSMSuSecRwStLegrestInOutPosDelta_Val/1 -> [KeSMSuSecRwStLegrestInOutPosDelta_Val]
  PA_KeSMSuSecRwStHeadrestUpwdDwnwdPosDelta_Val/1 -> [KeSMSuSecRwStHeadrestUpwdDwnwdPosDelta_Val]
  PA_KeSMSuSecRwStFtrstUpwdDnwdPosDelta_Val/1 -> [KeSMSuSecRwStFtrstUpwdDnwdPosDelta_Val]
  Bus Selector2/13 -> [K_FtrstUpwdPos]  "<FtrstUpwdDnwdPos>"
  Bus Selector2/14 -> [K_FtrstUpwdPosMax]  "<FtrstUpwdDnwdPosMax>"
  Bus Selector2/15 -> [K_FtrstUpwdPosMin]  "<FtrstUpwdDnwdPosMin>"
  Bus Selector2/12 -> [K_LgrstOtwdInwdPosMin]  "<LgrstOtwdInwdPosMin>"
  Bus Selector2/11 -> [K_LgrstOtwdInwdPosMax]  "<LgrstOtwdInwdPosMax>"
  Bus Selector2/10 -> [K_LgrstOtwdInwdPos]  "<LgrstOtwdInwdPos>"
  [LgrstUpwdMovConfig] -> SecRwLtStLgrstUpwd_Lt_Step3/14
  PA_KeSMSwDltTrgtPos_Val9/1 -> SecRwLtStLgrstUpwd_Lt_Step3/13
  Bus Selector4/1 -> [BkReclnUpwdDnwdMovConfig]  "<BkReclnUpwdDnwdMovConfig>"
  Bus Selector4/2 -> [ArmTouchMovConfig]  "<ArmTouchMovConfig>"
  Bus Selector4/4 -> [LgrstUpwdMovConfig]  "<LgrstUpwdMovConfig>"
  Bus Selector4/5 -> [LtwdRtwdMovConfig]  "<LtwdRtwdMovConfig>"
  Bus Selector4/3 -> [FrwdBkwdMovConfig]  "<FrwdBkwdMovConfig>"
  StConfig/1 -> Bus Selector4/1
  ModeStCalib_2L/1 -> Bus Selector3/1
  Bus Selector2/3 -> [K_BkReclnUpwdDnwdPosMin]  "<BkReclnUpwdDnwdPosMin>"
  Bus Selector3/1 -> Bus Selector2/1  "<LgrstOpenRSecRwRtSt>"
  Bus Selector2/2 -> [K_BkReclnUpwdDnwdPosMax]  "<BkReclnUpwdDnwdPosMax>"
  Bus Selector2/1 -> [K_BkReclnUpwdDnwdPos]  "<BkReclnUpwdDnwdPos>"
  Bus Selector2/4 -> [K_HdrstUpwdPos]  "<HdrstUpwdPos>"
  Bus Selector2/8 -> [K_LgrstUpwdPosMax]  "<LgrstUpwdPosMax>"
  Bus Selector2/5 -> [K_HdrstUpwdPosMax]  "<HdrstUpwdPosMax>"
  Bus Selector2/7 -> [K_LgrstUpwdPos]  "<LgrstUpwdPos>"
  Bus Selector2/6 -> [K_HdrstUpwdPosMin]  "<HdrstUpwdPosMin>"
  Bus Selector2/9 -> [K_LgrstUpwdPosMin]  "<LgrstUpwdPosMin>"
  Bus Selector1/6 -> [R2LtStArmScrnPosV]  "<SecRwRtStArmScrnPosV_Val_read>"
  [KeSMSuMdMotFinshdTm_Val] -> SecRwLtStLgrstUpwd_Lt_Step3/12
  PA_KeSMSuMdMotFinshdTm_Val/1 -> [KeSMSuMdMotFinshdTm_Val]
  PA_KeSMSuSecRwStLegrestUpwdDwnwdPosDelta_Val/1 -> [KeSMSuSecRwStLegrestUpwdDwnwdPosDelta_Val]
  PA_KeSMSuSecRwStBackPosDelta_Val/1 -> [KeSMSuSecRwStBackPosDelta_Val]
  PA_KeSMSwDltTrgtPos_Val7/1 -> Bus Creator/9  "SecRwRtStArmScrnTrgtPos"
  PA_KeSMSuModeReqDurgTm_Val/1 -> [Tick]
  PA_KeSMSwDltTrgtPos_Val20/1 -> Bus Creator/4  "SecRwRtStCshnRrUpwdDnwdTrgtPos"
  PA_KeSMSwDltTrgtPos_Val8/1 -> Bus Creator/5  "SecRwRtStFrwdBkwdTrgtPos"
  PA_KeSMSwDltTrgtPos_Val5/1 -> Bus Creator/1  "SecRwRtStBkReclnUpwdDnwdTrgtPos"
  PA_KeSMSwDltTrgtPos_Val18/1 -> Bus Creator/2  "SecRwRtStBlstOtwdInwdTrgtPos"
  PA_KeSMSwDltTrgtPos_Val1/1 -> Bus Creator/8  "SecRwRtStLtwdRtwdTrgtPos"
  PA_KeSMSwDltTrgtPos_Val19/1 -> Bus Creator/3  "SecRwRtStCshnFrntUpwdDnwdTrgtPos"
  [R2Lt_LgrstUpwd_TarPos] -> Bus Creator/7  "SecRwRtStLgrstUpwdDnwdTrgtPos"
  Bus Creator/1 -> R2Rt_TrgtPoss/1
  PA_KeSMSwDltTrgtPos_Val3/1 -> Bus Creator/6  "SecRwRtStHdrstUpwdDnwdTrgtPos"
  SecRwLtStLgrstUpwd_Lt_Step3/4 -> [lgrstStep1_done]
  SecRwLtStLgrstUpwd_Lt_Step3/3 -> [R2Lt_LgrstUpwd_TarPos]
  SecRwLtStLgrstUpwd_Lt_Step3/2 -> [lgrst_ArrivedTarPos]
  [Tick] -> SecRwLtStLgrstUpwd_Lt_Step3/11
  PA_KeSMSwDltTrgtPos_Val12/1 -> SecRwLtStLgrstUpwd_Lt_Step3/10
  PA_KeSMSwDltTrgtPos_Val10/1 -> SecRwLtStLgrstUpwd_Lt_Step3/9
  [SecRwLtStLgrstUpwdDnwdPosV] -> SecRwLtStLgrstUpwd_Lt_Step3/8
  [KeSMSuSecRwStLegrestUpwdDwnwdPosDelta_Val] -> SecRwLtStLgrstUpwd_Lt_Step3/7
  [SecRwLtStLgrstUpwdDnwdPos] -> SecRwLtStLgrstUpwd_Lt_Step3/3
  [K_LgrstUpwdPos] -> SecRwLtStLgrstUpwd_Lt_Step3/6
  [K_LgrstUpwdPosMax] -> SecRwLtStLgrstUpwd_Lt_Step3/5
  [K_LgrstUpwdPosMin] -> SecRwLtStLgrstUpwd_Lt_Step3/4
  [StepEn_LgrstStep1] -> SecRwLtStLgrstUpwd_Lt_Step3/2
  [Trig] -> SecRwLtStLgrstUpwd_Lt_Step3/1
  Bus Selector/1 -> [SecRwLtStBkReclnUpwdDnwdPos]  "<IfVeSMSuSecRwRtStBkReclnUpwdDnwdPos_Val_read>"
  Bus Selector1/2 -> [SecRwLtStFrwdBkwdPosV]  "<IfVeSMSuSecRwRtStFrwdBkwdPosV_Val_read>"
  Bus Selector1/1 -> [SecRwLtStBkReclnUpwdDnwdPosV]  "<IfVeSMSuSecRwRtStBkReclnUpwdDnwdPosV_Val_read>"
  Bus Selector1/5 -> [SecRwLtStLtwdRtwdPosV]  "<IfVeSMSuSecRwRtStLtwdRtwdPosV_Val_read>"
  SecRwLtStPossV/1 -> Bus Selector1/1
  Bus Selector1/4 -> [SecRwLtStLgrstUpwdDnwdPosV]  "<IfVeSMSuSecRwRtStLgrstUpwdDnwdPosV_Val_read>"
  SecRwLtStsPoss/1 -> Bus Selector/1
  Bus Selector1/3 -> [SecRwLtStHPassStUpwdDnwdPosV]  "<IfVeSMSuSecRwRtStHPassStUpwdDnwdPosV_Val_read>"
  Mode_Trig/1 -> [Trig]
  SecRwLtStLgrstUpwd_Lt_Step3/1 -> [lgrstStep1_ini]
  PA_KeSMSwDltTrgtPos_Val4/1 -> IfVeSMSuSecRwLtStRclCmdSrv_Val_writeRaw/1
  [CntLow] -> SecRwLtStFtUpwd_Lt_Step2/15
  [CntLow] -> SecRwLtStLgrstOtwd_Lt_Step1/15
  [CntLow] -> SecRwLtStLgrstUpwd_Lt_Step3/15
  PA_KeSMSuMdRetryTm1_Val/1 -> [CntLow]
  PA_KeSMSwDltTrgtPos_Val6/1 -> Bus Creator1/3  "SecRwRtStHdrstFrwdBkwdTrgtPos"
  Bus Selector7/4 -> [HdrstFrwdBkwdMovConfig]  "<HdrstFrwdBkwdMovConfig>"
  Bus Selector5/3 -> [SecRwLtStHdrstFrwdBkwdPos]  "<IfVeSMSuSecRwRtStHdrstFrwdBkwdPos_Val_read>"
  Bus Selector6/3 -> [SecRwLtStHdrstFrwdBkwdPosV]  "<IfVeSMSuSecRwRtStHdrstFrwdBkwdPosV_Val_read>"
  Bus Selector2/16 -> [K_HdrstFrwdBkwdnwdPos]  "<HdrstFrwdBkwdnwdPos>"
  Bus Selector2/17 -> [K_HdrstFrwdBkwdnwdPosMax]  "<HdrstFrwdBkwdnwdPosMax>"
  Bus Selector2/18 -> [K_HdrstFrwdBkwdnwdPosMin]  "<HdrstFrwdBkwdnwdPosMin>"
  PA_KeSMSuSecRwStHeadrestFwdBkwdPosDelta_Val/1 -> [KeSMSuSecRwStHeadrestFwdBkwdPosDelta_Val]
  Bus Selector/6 -> [R2LtStArmScrnPos]  "<SecRwRtStArmScrnPos_Val_read>"
  Bus Selector/5 -> [SecRwLtStLtwdRtwdPos]  "<IfVeSMSuSecRwRtStLtwdRtwdPos_Val_read>"
  Bus Selector/4 -> [SecRwLtStLgrstUpwdDnwdPos]  "<IfVeSMSuSecRwRtStLgrstUpwdDnwdPos_Val_read>"
  Bus Selector/3 -> [SecRwLtStHPassStUpwdDnwdPos]  "<IfVeSMSuSecRwRtStHPassStUpwdDnwdPos_Val_read>"
  Bus Selector/2 -> [SecRwLtStFrwdBkwdPos]  "<IfVeSMSuSecRwRtStFrwdBkwdPos_Val_read>"

== system ModeAdjust/ModeAdjustRunnable_sys/ModeAdjust/LugL/R3Lt ==
  Mode_Trig : Inport
  Step1En : Inport  Port=2
  Step2En : Inport  Port=3
  isSeatOccupied : Inport  Port=4
  ThdRwLtStPoss : Inport  Port=5
  ThdRwLtStPossV : Inport  Port=6
  ModeStCalib_3L : Inport  Port=7
  is6s : Inport  Port=8
  StConfig : Inport  Port=9
  ThdRwLtStFrwdCmdSrv : Inport  Port=10
  Bus Creator : BusCreator  Inputs=3  OutDataTypeStr=Bus: ThdRwLfSeatPos
  Bus Selector : BusSelector  OutputSignals=IfVeSMSuThdRwLtStBkReclnUpwdDnwdPos_Val_read,IfVeSMSuThdRwLtStCshnFldUpwdDnwdPos_Val_read,IfVeSMSuThdRwLtStFrwdBkwdPos_Val_read
  Bus Selector1 : BusSelector  OutputSignals=IfVeSMSuThdRwLtStBkReclnUpwdDnwdPosV_Val_read,IfVeSMSuThdRwLtStCshnFldUpwdDnwdPosV_Val_read,IfVeSMSuThdRwLtStFrwdBkwdPosV_Val_read
  Bus Selector2 : BusSelector  OutputSignals=BkReclnUpwdDnwdPos,BkReclnUpwdDnwdPosMax,BkReclnUpwdDnwdPosMin,CshnFldUpwdDnwdPos,CshnFldUpwdDnwdPosMax,CshnFldUpwdDnwdPosMin,FrwdBkwdPos,FrwdBkwdPosMax,FrwdBkwdPosMin
  Bus Selector3 : BusSelector  OutputSignals=LugThdRwLtSt
  Bus Selector4 : BusSelector  OutputSignals=BkReclnUpwdDnwdMovConfig,CshnFldUpwdDnwdMovConfig,FrwdBkwdMovConfig
  Constant : Constant  Value=3  OutDataTypeStr=uint8
  Constant1 : Constant  Value=0  OutDataTypeStr=uint8
  Delay1 : Delay  DelayLength=1
  Delay2 : Delay  DelayLength=1
  Logical Operator{,4,9,13} (4 alike) : Logic  AllPortsSameDT=off  OutDataTypeStr=boolean
  Logical Operator5 : Logic  Operator=OR  AllPortsSameDT=off  OutDataTypeStr=boolean
  Logical Operator6 : Logic  Operator=OR  AllPortsSameDT=off  OutDataTypeStr=boolean
  NOT : Logic  Operator=NOT  AllPortsSameDT=off  OutDataTypeStr=boolean
  PA_KeSMSuMdMotFinshdTm_Val : Constant  Value=KeSMSuMdMotFinshdTm_Val
  PA_KeSMSuMdRetryTm1_Val : Constant  Value=KeSMSuMdRetryTm1_Val
  PA_KeSMSuModeReqDurgTm_Val : Constant  Value=KeSMSuModeReqDurgTm_Val
  PA_KeSMSuThirdRwStFwdBkwdPosDelta_Val : Constant  Value=KeSMSuThirdRwStFwdBkwdPosDelta_Val
  PA_KeSMSuThrdRwCushFoldPosDelta_Val : Constant  Value=KeSMSuThrdRwCushFoldPosDelta_Val
  PA_KeSMSuThrdRwStBackPosDelta_Val : Constant  Value=KeSMSuThrdRwStBackPosDelta_Val
  PA_KeSMSwDltTrgtPos_Val{3,6..7,18} (4 alike) : Constant  Value=KeSMSwPosInvalidVal_Val
  PA_KeSMSwDltTrgtPos_Val24 : Constant  OutDataTypeStr=boolean
  PA_KeSMSwDltTrgtPos_Val5 : Constant  Value=0  OutDataTypeStr=boolean
  R3LtSt_BkReclnUpwdDnwd_Step1 : Lib/CommonUsed  SystemSampleTime=-1
  R3LtSt_CshnFldUpwdDnwd_Step3 : Lib/CommonUsed  SystemSampleTime=-1
  R3LtSt_FrwdBkwd_Step2 : Lib/CommonUsed  SystemSampleTime=-1
  Relational Operator1 : RelationalOperator  Operator=~=  OutDataTypeStr=boolean  RndMeth=Simplest
  Switch : Switch  Criteria=u2 ~= 0
  R3Lt_Step1_ini : Outport
  R3Lt_Step2_ini : Outport  Port=2
  R3Lt_Step1done : Outport  Port=3
  R3Lt_Step2done : Outport  Port=4
  IfVeSMSbThdRwLtStRclCmdSrv_Val_writeRaw : Outport  Port=5
  R3Lt_TrgtPoss : Outport  Port=6  VectorParamsAs1DForOutWhenUnconnected=on
  R3Lt_All_done : Outport  Port=7
  R3Lt_SpdCtrl : Outport  Port=8  VectorParamsAs1DForOutWhenUnconnected=on
  wires:
  Bus Creator/1 -> R3Lt_TrgtPoss/1
  [R3Lt_BkReclnUpwdDnwd_TarPos] -> Bus Creator/1  "ThdRwLtStBkReclnUpwdDnwdTrgtPos"
  [R3Lt_CshnFldUpwdDnwd_TarPos] -> Bus Creator/2  "ThdRwLtStCshnFldUpwdDnwdTrgtPos"
  [R3LtFrwdBkwd_TarPos] -> Bus Creator/3  "ThdRwLtStFrwdBkwdTrgtPos"
  Bus Selector/1 -> [ThdRwLtStBkReclnUpwdDnwdPos]  "<IfVeSMSuThdRwLtStBkReclnUpwdDnwdPos_Val_read>"
  Bus Selector1/1 -> [ThdRwLtStBkReclnUpwdDnwdPosV]  "<IfVeSMSuThdRwLtStBkReclnUpwdDnwdPosV_Val_read>"
  ThdRwLtStPossV/1 -> Bus Selector1/1
  Bus Selector1/3 -> [ThdRwLtStFrwdBkwdPosV]  "<IfVeSMSuThdRwLtStFrwdBkwdPosV_Val_read>"
  Bus Selector/3 -> [ThdRwLtStFrwdBkwdPos]  "<IfVeSMSuThdRwLtStFrwdBkwdPos_Val_read>"
  ThdRwLtStPoss/1 -> Bus Selector/1
  Bus Selector1/2 -> [ThdRwLtStCshnFldUpwdDnwdPosV]  "<IfVeSMSuThdRwLtStCshnFldUpwdDnwdPosV_Val_read>"
  Bus Selector/2 -> [ThdRwLtStCshnFldUpwdDnwdPos]  "<IfVeSMSuThdRwLtStCshnFldUpwdDnwdPos_Val_read>"
  [K_BkReclnUpwdDnwdPosMax] -> R3LtSt_BkReclnUpwdDnwd_Step1/5
  [Trig] -> R3LtSt_BkReclnUpwdDnwd_Step1/1
  R3LtSt_CshnFldUpwdDnwd_Step3/2 -> [Step3ArrivedTarPos]
  Mode_Trig/1 -> [Trig]
  [K_CshnFldUpwdDnwdPosMax] -> R3LtSt_CshnFldUpwdDnwd_Step3/5
  [KeSMSuThrdRwStBackPosDelta_Val] -> R3LtSt_BkReclnUpwdDnwd_Step1/7
  [ThdRwLtStFrwdBkwdPos] -> R3LtSt_FrwdBkwd_Step2/3
  [ThdRwLtStCshnFldUpwdDnwdPos] -> R3LtSt_CshnFldUpwdDnwd_Step3/3
  [K_FrwdBkwdPosMax] -> R3LtSt_FrwdBkwd_Step2/5
  R3LtSt_CshnFldUpwdDnwd_Step3/1 -> [R3Lt_Step1_2_ini]
  [K_CshnFldUpwdDnwdPos] -> R3LtSt_CshnFldUpwdDnwd_Step3/6
  [KeSMSuThirdRwStFwdBkwdPosDelta_Val] -> R3LtSt_FrwdBkwd_Step2/7
  [K_FrwdBkwdPosMin] -> R3LtSt_FrwdBkwd_Step2/4
  [KeSMSuThrdRwCushFoldPosDelta_Val] -> R3LtSt_CshnFldUpwdDnwd_Step3/7
  R3LtSt_FrwdBkwd_Step2/2 -> [Step2ArrivedTarPos]
  [K_BkReclnUpwdDnwdPosMin] -> R3LtSt_BkReclnUpwdDnwd_Step1/4
  R3LtSt_BkReclnUpwdDnwd_Step1/2 -> [Step1ArrivedTarPos]
  [ThdRwLtStBkReclnUpwdDnwdPos] -> R3LtSt_BkReclnUpwdDnwd_Step1/3
  [K_CshnFldUpwdDnwdPosMin] -> R3LtSt_CshnFldUpwdDnwd_Step3/4
  [K_BkReclnUpwdDnwdPos] -> R3LtSt_BkReclnUpwdDnwd_Step1/6
  [ThdRwLtStBkReclnUpwdDnwdPosV] -> R3LtSt_BkReclnUpwdDnwd_Step1/8
  PA_KeSMSwDltTrgtPos_Val3/1 -> R3LtSt_BkReclnUpwdDnwd_Step1/10
  R3LtSt_BkReclnUpwdDnwd_Step1/3 -> [R3Lt_BkReclnUpwdDnwd_TarPos]
  R3LtSt_BkReclnUpwdDnwd_Step1/4 -> [Step1_1_done]
  Step1En/1 -> R3LtSt_BkReclnUpwdDnwd_Step1/2, [Step1En]
  [Trig] -> R3LtSt_FrwdBkwd_Step2/1
  [K_FrwdBkwdPos] -> R3LtSt_FrwdBkwd_Step2/6
  [ThdRwLtStFrwdBkwdPosV] -> R3LtSt_FrwdBkwd_Step2/8
  isSeatOccupied/1 -> [isSeatOccupied]
  [isSeatOccupied] -> R3LtSt_BkReclnUpwdDnwd_Step1/9
  [isSeatOccupied] -> R3LtSt_FrwdBkwd_Step2/9
  PA_KeSMSwDltTrgtPos_Val6/1 -> R3LtSt_FrwdBkwd_Step2/10
  [Tick] -> R3LtSt_BkReclnUpwdDnwd_Step1/11
  [Tick] -> R3LtSt_FrwdBkwd_Step2/11
  R3LtSt_FrwdBkwd_Step2/3 -> [R3LtFrwdBkwd_TarPos]
  R3LtSt_FrwdBkwd_Step2/4 -> [Step2_done]
  [Trig] -> R3LtSt_CshnFldUpwdDnwd_Step3/1
  [isSeatOccupied] -> R3LtSt_CshnFldUpwdDnwd_Step3/9
  PA_KeSMSwDltTrgtPos_Val7/1 -> R3LtSt_CshnFldUpwdDnwd_Step3/10
  [Tick] -> R3LtSt_CshnFldUpwdDnwd_Step3/11
  [ThdRwLtStCshnFldUpwdDnwdPosV] -> R3LtSt_CshnFldUpwdDnwd_Step3/8
  R3LtSt_CshnFldUpwdDnwd_Step3/3 -> [R3Lt_CshnFldUpwdDnwd_TarPos]
  Logical Operator4/1 -> Delay2/1
  R3LtSt_BkReclnUpwdDnwd_Step1/1 -> [R3Lt_Step1_1_ini]
  Logical Operator/1 -> Logical Operator6/1, R3Lt_Step1_ini/1
  Logical Operator6/1 -> R3Lt_Step1done/1, [R3Lt_Step1_done]
  Logical Operator13/1 -> Delay1/1
  R3LtSt_CshnFldUpwdDnwd_Step3/4 -> [R3Lt_Step1_2_done]
  [R3Lt_Step1_done] -> Logical Operator13/1
  Delay1/1 -> Logical Operator5/2
  Delay2/1 -> Logical Operator6/2
  [R3Lt_Step1_1_ini] -> Logical Operator/1
  [R3Lt_Step1_2_ini] -> Logical Operator/2
  R3LtSt_FrwdBkwd_Step2/1 -> [Step2_ini_done], R3Lt_Step2_ini/1
  PA_KeSMSwDltTrgtPos_Val24/1 -> IfVeSMSbThdRwLtStRclCmdSrv_Val_writeRaw/1
  [Step1_1_done] -> Logical Operator4/1
  [R3Lt_Step1_2_done] -> Logical Operator4/2
  [Step2_done] -> Logical Operator13/2
  [Step1En] -> R3LtSt_CshnFldUpwdDnwd_Step3/2
  Step2En/1 -> R3LtSt_FrwdBkwd_Step2/2
  [Step2_ini_done] -> Logical Operator5/1
  Logical Operator5/1 -> Logical Operator9/1, R3Lt_Step2done/1
  Logical Operator9/1 -> R3Lt_All_done/1
  [R3Lt_Step1_done] -> Logical Operator9/2
  PA_KeSMSuModeReqDurgTm_Val/1 -> [Tick]
  PA_KeSMSuMdMotFinshdTm_Val/1 -> [KeSMSuMdMotFinshdTm_Val]
  PA_KeSMSuThrdRwCushFoldPosDelta_Val/1 -> [KeSMSuThrdRwCushFoldPosDelta_Val]
  PA_KeSMSuThirdRwStFwdBkwdPosDelta_Val/1 -> [KeSMSuThirdRwStFwdBkwdPosDelta_Val]
  PA_KeSMSuThrdRwStBackPosDelta_Val/1 -> [KeSMSuThrdRwStBackPosDelta_Val]
  [KeSMSuMdMotFinshdTm_Val] -> R3LtSt_BkReclnUpwdDnwd_Step1/12
  [KeSMSuMdMotFinshdTm_Val] -> R3LtSt_FrwdBkwd_Step2/12
  [KeSMSuMdMotFinshdTm_Val] -> R3LtSt_CshnFldUpwdDnwd_Step3/12
  Bus Selector2/6 -> [K_CshnFldUpwdDnwdPosMin]  "<CshnFldUpwdDnwdPosMin>"
  Bus Selector2/4 -> [K_CshnFldUpwdDnwdPos]  "<CshnFldUpwdDnwdPos>"
  Bus Selector2/7 -> [K_FrwdBkwdPos]  "<FrwdBkwdPos>"
  Bus Selector2/5 -> [K_CshnFldUpwdDnwdPosMax]  "<CshnFldUpwdDnwdPosMax>"
  ModeStCalib_3L/1 -> Bus Selector3/1
  Bus Selector2/3 -> [K_BkReclnUpwdDnwdPosMin]  "<BkReclnUpwdDnwdPosMin>"
  Bus Selector3/1 -> Bus Selector2/1  "<LugThdRwLtSt>"
  Bus Selector2/9 -> [K_FrwdBkwdPosMin]  "<FrwdBkwdPosMin>"
  Bus Selector2/2 -> [K_BkReclnUpwdDnwdPosMax]  "<BkReclnUpwdDnwdPosMax>"
  Bus Selector2/1 -> [K_BkReclnUpwdDnwdPos]  "<BkReclnUpwdDnwdPos>"
  Bus Selector2/8 -> [K_FrwdBkwdPosMax]  "<FrwdBkwdPosMax>"
  [is6s] -> R3LtSt_CshnFldUpwdDnwd_Step3/13
  is6s/1 -> [is6s]
  NOT/1 -> R3LtSt_FrwdBkwd_Step2/13
  PA_KeSMSwDltTrgtPos_Val5/1 -> R3LtSt_BkReclnUpwdDnwd_Step1/13
  Bus Selector4/1 -> [BkReclnUpwdDnwdMovConfig]  "<BkReclnUpwdDnwdMovConfig>"
  StConfig/1 -> Bus Selector4/1
  Bus Selector4/2 -> [CshnFldUpwdDnwdMovConfig]  "<CshnFldUpwdDnwdMovConfig>"
  Bus Selector4/3 -> [FrwdBkwdMovConfig]  "<FrwdBkwdMovConfig>"
  [CshnFldUpwdDnwdMovConfig] -> R3LtSt_CshnFldUpwdDnwd_Step3/14
  [FrwdBkwdMovConfig] -> R3LtSt_FrwdBkwd_Step2/14
  [BkReclnUpwdDnwdMovConfig] -> R3LtSt_BkReclnUpwdDnwd_Step1/14
  [CntLow] -> R3LtSt_BkReclnUpwdDnwd_Step1/15
  [CntLow] -> R3LtSt_CshnFldUpwdDnwd_Step3/15
  PA_KeSMSuMdRetryTm1_Val/1 -> [CntLow]
  [CntLow] -> R3LtSt_FrwdBkwd_Step2/15
  [R3LtFrwdBkwd_TarPos] -> Relational Operator1/1  "ThdRwLtStFrwdBkwdTrgtPos"
  Switch/1 -> R3Lt_SpdCtrl/1
  Relational Operator1/1 -> Switch/2
  Constant/1 -> Switch/1
  Constant1/1 -> Switch/3
  PA_KeSMSwDltTrgtPos_Val18/1 -> Relational Operator1/2
  ThdRwLtStFrwdCmdSrv/1 -> NOT/1

== system ModeAdjust/ModeAdjustRunnable_sys/ModeAdjust/LugR/R3Rt ==
  Mode_Trig : Inport
  Step1En : Inport  Port=2
  Step2En : Inport  Port=3
  SeatOccupied : Inport  Port=4
  ThdRwRtStPoss : Inport  Port=5
  ThdRwRtStPossV : Inport  Port=6
  ModeStCalib_3R : Inport  Port=7
  is6s : Inport  Port=8
  StConfig : Inport  Port=9
  ThdRwRtStFrwdCmdSrv : Inport  Port=10
  Bus Creator : BusCreator  Inputs=3  OutDataTypeStr=Bus: ThdRwRtSeatPos
  Bus Selector : BusSelector  OutputSignals=IfVeSMSuThdRwRtStBkReclnUpwdDnwdPos_Val_read,IfVeSMSuThdRwRtStCshnFldUpwdDnwdPos_Val_read,IfVeSMSuThdRwRtStFrwdBkwdPos_Val_read
  Bus Selector1 : BusSelector  OutputSignals=IfVeSMSuThdRwRtStBkReclnUpwdDnwdPosV_Val_read,IfVeSMSuThdRwRtStCshnFldUpwdDnwdPosV_Val_read,IfVeSMSuThdRwRtStFrwdBkwdPosV_Val_read
  Bus Selector2 : BusSelector  OutputSignals=BkReclnUpwdDnwdPos,BkReclnUpwdDnwdPosMax,BkReclnUpwdDnwdPosMin,CshnFldUpwdDnwdPos,CshnFldUpwdDnwdPosMax,CshnFldUpwdDnwdPosMin,FrwdBkwdPos,FrwdBkwdPosMax,FrwdBkwdPosMin
  Bus Selector3 : BusSelector  OutputSignals=LugThdRwRtSt
  Bus Selector4 : BusSelector  OutputSignals=BkReclnUpwdDnwdMovConfig,CshnFldUpwdDnwdMovConfig,FrwdBkwdMovConfig
  Constant : Constant  Value=3  OutDataTypeStr=uint8
  Constant1 : Constant  Value=0  OutDataTypeStr=uint8
  Delay1 : Delay  DelayLength=1
  Logical Operator{,4,8..9} (4 alike) : Logic  AllPortsSameDT=off  OutDataTypeStr=boolean
  Logical Operator5 : Logic  Operator=OR  AllPortsSameDT=off  OutDataTypeStr=boolean
  Logical Operator6 : Logic  Operator=OR  AllPortsSameDT=off  OutDataTypeStr=boolean
  NOT : Logic  Operator=NOT  AllPortsSameDT=off  OutDataTypeStr=boolean
  PA_KeSMSuMdMotFinshdTm_Val : Constant  Value=KeSMSuMdMotFinshdTm_Val
  PA_KeSMSuMdRetryTm1_Val : Constant  Value=KeSMSuMdRetryTm1_Val
  PA_KeSMSuModeReqDurgTm_Val : Constant  Value=KeSMSuModeReqDurgTm_Val
  PA_KeSMSuThirdRwStFwdBkwdPosDelta_Val : Constant  Value=KeSMSuThirdRwStFwdBkwdPosDelta_Val
  PA_KeSMSuThrdRwCushFoldPosDelta_Val : Constant  Value=KeSMSuThrdRwCushFoldPosDelta_Val
  PA_KeSMSuThrdRwStBackPosDelta_Val : Constant  Value=KeSMSuThrdRwStBackPosDelta_Val
  PA_KeSMSwDltTrgtPos_Val{3,6..7,18} (4 alike) : Constant  Value=KeSMSwPosInvalidVal_Val
  PA_KeSMSwDltTrgtPos_Val2 : Constant  Value=0  OutDataTypeStr=boolean
  PA_KeSMSwDltTrgtPos_Val9 : Constant  OutDataTypeStr=boolean
  R3RtReclnUpDn_Step1 : Lib/CommonUsed  SystemSampleTime=-1
  R3RtReclnUpDn_Step2 : Lib/CommonUsed  SystemSampleTime=-1
  R3Rt_CshnFldUpwdDnwd_Step1 : Lib/CommonUsed  SystemSampleTime=-1
  Relational Operator1 : RelationalOperator  Operator=~=  OutDataTypeStr=boolean  RndMeth=Simplest
  Switch : Switch  Criteria=u2 ~= 0
  Unit Delay : UnitDelay  SampleTime=-1
  R3Rt_Step1_ini : Outport
  R3Rt_Step2_ini : Outport  Port=2
  R3Rt_Step1done : Outport  Port=3
  R3Rt_Step2_done : Outport  Port=4
  IfVeSMSbThdRwRtStRclCmdSrv_Val_writeRaw : Outport  Port=5
  R3Rt_TrgtPoss : Outport  Port=6  VectorParamsAs1DForOutWhenUnconnected=on
  R3Rt_All_done : Outport  Port=7
  R3Lt_SpdCtrl : Outport  Port=8  VectorParamsAs1DForOutWhenUnconnected=on
  wires:
  PA_KeSMSwDltTrgtPos_Val2/1 -> R3RtReclnUpDn_Step1/13
  NOT/1 -> R3RtReclnUpDn_Step2/13
  is6s/1 -> [is6s]
  [is6s] -> R3Rt_CshnFldUpwdDnwd_Step1/13
  Bus Selector2/8 -> [K_FrwdBkwdPosMax]  "<FrwdBkwdPosMax>"
  Bus Selector2/1 -> [K_BkReclnUpwdDnwdPos]  "<BkReclnUpwdDnwdPos>"
  Bus Selector2/2 -> [K_BkReclnUpwdDnwdPosMax]  "<BkReclnUpwdDnwdPosMax>"
  Bus Selector2/9 -> [K_FrwdBkwdPosMin]  "<FrwdBkwdPosMin>"
  Bus Selector3/1 -> Bus Selector2/1  "<LugThdRwRtSt>"
  Bus Selector2/3 -> [K_BkReclnUpwdDnwdPosMin]  "<BkReclnUpwdDnwdPosMin>"
  ModeStCalib_3R/1 -> Bus Selector3/1
  Bus Selector2/5 -> [K_CshnFldUpwdDnwdPosMax]  "<CshnFldUpwdDnwdPosMax>"
  Bus Selector2/7 -> [K_FrwdBkwdPos]  "<FrwdBkwdPos>"
  Bus Selector2/4 -> [K_CshnFldUpwdDnwdPos]  "<CshnFldUpwdDnwdPos>"
  Bus Selector2/6 -> [K_CshnFldUpwdDnwdPosMin]  "<CshnFldUpwdDnwdPosMin>"
  [KeSMSuMdMotFinshdTm_Val] -> R3Rt_CshnFldUpwdDnwd_Step1/12
  [KeSMSuMdMotFinshdTm_Val] -> R3RtReclnUpDn_Step2/12
  [KeSMSuMdMotFinshdTm_Val] -> R3RtReclnUpDn_Step1/12
  PA_KeSMSuThrdRwStBackPosDelta_Val/1 -> [KeSMSuThrdRwStBackPosDelta_Val]
  PA_KeSMSuThirdRwStFwdBkwdPosDelta_Val/1 -> [KeSMSuThirdRwStFwdBkwdPosDelta_Val]
  PA_KeSMSuThrdRwCushFoldPosDelta_Val/1 -> [KeSMSuThrdRwCushFoldPosDelta_Val]
  PA_KeSMSuMdMotFinshdTm_Val/1 -> [KeSMSuMdMotFinshdTm_Val]
  PA_KeSMSuModeReqDurgTm_Val/1 -> [Tick]
  Logical Operator9/1 -> R3Rt_All_done/1
  [R3Rt__Step1done] -> Logical Operator9/2
  [Step2_done] -> Logical Operator8/2
  Step2En/1 -> R3RtReclnUpDn_Step2/2
  [Step1En] -> R3Rt_CshnFldUpwdDnwd_Step1/2
  [R3Rt__Step1done] -> Logical Operator8/1
  [R3Rt_Step2_done] -> Logical Operator4/2
  [Step1_1_done] -> Logical Operator4/1
  [R3Rt_Step1_2_ini] -> Logical Operator/2
  [R3Rt_Step1_1_ini] -> Logical Operator/1
  PA_KeSMSwDltTrgtPos_Val9/1 -> IfVeSMSbThdRwRtStRclCmdSrv_Val_writeRaw/1
  Logical Operator6/1 -> [R3Rt__Step1done], R3Rt_Step1done/1
  [R3Rt_Step2_ini] -> Logical Operator5/1
  Delay1/1 -> Logical Operator5/2
  Logical Operator5/1 -> R3Rt_Step2_done/1, Logical Operator9/1
  Logical Operator8/1 -> Delay1/1
  R3Rt_CshnFldUpwdDnwd_Step1/4 -> [R3Rt_Step2_done]
  Unit Delay/1 -> Logical Operator6/2
  Logical Operator4/1 -> Unit Delay/1
  Logical Operator/1 -> R3Rt_Step1_ini/1, Logical Operator6/1
  R3RtReclnUpDn_Step1/1 -> [R3Rt_Step1_1_ini]
  [K_BkReclnUpwdDnwdPosMax] -> R3RtReclnUpDn_Step1/5
  [Trig] -> R3RtReclnUpDn_Step1/1
  R3Rt_CshnFldUpwdDnwd_Step1/2 -> [Step3ArrivedTarPos]
  Mode_Trig/1 -> [Trig]
  [K_CshnFldUpwdDnwdPosMax] -> R3Rt_CshnFldUpwdDnwd_Step1/5
  [KeSMSuThrdRwStBackPosDelta_Val] -> R3RtReclnUpDn_Step1/7
  [ThdRwRtStFrwdBkwdPos] -> R3RtReclnUpDn_Step2/3
  [ThdRwRtStCshnFldUpwdDnwdPos] -> R3Rt_CshnFldUpwdDnwd_Step1/3
  [K_FrwdBkwdPosMax] -> R3RtReclnUpDn_Step2/5
  R3Rt_CshnFldUpwdDnwd_Step1/1 -> [R3Rt_Step1_2_ini]
  [K_CshnFldUpwdDnwdPos] -> R3Rt_CshnFldUpwdDnwd_Step1/6
  [KeSMSuThirdRwStFwdBkwdPosDelta_Val] -> R3RtReclnUpDn_Step2/7
  [K_FrwdBkwdPosMin] -> R3RtReclnUpDn_Step2/4
  [KeSMSuThrdRwCushFoldPosDelta_Val] -> R3Rt_CshnFldUpwdDnwd_Step1/7
  R3RtReclnUpDn_Step2/1 -> R3Rt_Step2_ini/1, [R3Rt_Step2_ini]
  R3RtReclnUpDn_Step2/2 -> [Step2ArrivedTarPos]
  [K_BkReclnUpwdDnwdPosMin] -> R3RtReclnUpDn_Step1/4
  R3RtReclnUpDn_Step1/2 -> [Step1ArrivedTarPos]
  [ThdRwRtStBkReclnUpwdDnwdPos] -> R3RtReclnUpDn_Step1/3
  [K_CshnFldUpwdDnwdPosMin] -> R3Rt_CshnFldUpwdDnwd_Step1/4
  [K_BkReclnUpwdDnwdPos] -> R3RtReclnUpDn_Step1/6
  [ThdRwRtStBkReclnUpwdDnwdPosV] -> R3RtReclnUpDn_Step1/8
  PA_KeSMSwDltTrgtPos_Val3/1 -> R3RtReclnUpDn_Step1/10
  R3RtReclnUpDn_Step1/3 -> [R3RtReclnUpDn_TarPos]
  R3RtReclnUpDn_Step1/4 -> [Step1_1_done]
  Step1En/1 -> [Step1En], R3RtReclnUpDn_Step1/2
  [Trig] -> R3RtReclnUpDn_Step2/1
  [K_FrwdBkwdPos] -> R3RtReclnUpDn_Step2/6
  [ThdRwRtStFrwdBkwdPosV] -> R3RtReclnUpDn_Step2/8
  SeatOccupied/1 -> [isSeatOccupied]
  [isSeatOccupied] -> R3RtReclnUpDn_Step1/9
  [isSeatOccupied] -> R3RtReclnUpDn_Step2/9
  PA_KeSMSwDltTrgtPos_Val6/1 -> R3RtReclnUpDn_Step2/10
  [Tick] -> R3RtReclnUpDn_Step1/11
  [Tick] -> R3RtReclnUpDn_Step2/11
  R3RtReclnUpDn_Step2/3 -> [R3Rt_FrwdBkwd_TarPos]
  R3RtReclnUpDn_Step2/4 -> [Step2_done]
  [Trig] -> R3Rt_CshnFldUpwdDnwd_Step1/1
  [isSeatOccupied] -> R3Rt_CshnFldUpwdDnwd_Step1/9
  PA_KeSMSwDltTrgtPos_Val7/1 -> R3Rt_CshnFldUpwdDnwd_Step1/10
  [Tick] -> R3Rt_CshnFldUpwdDnwd_Step1/11
  [ThdRwRtStCshnFldUpwdDnwdPosV] -> R3Rt_CshnFldUpwdDnwd_Step1/8
  R3Rt_CshnFldUpwdDnwd_Step1/3 -> [R3Rt_CshnFldUpwdDnwd_TarPos]
  Bus Selector1/1 -> [ThdRwRtStBkReclnUpwdDnwdPosV]  "<IfVeSMSuThdRwRtStBkReclnUpwdDnwdPosV_Val_read>"
  Bus Selector/3 -> [ThdRwRtStFrwdBkwdPos]  "<IfVeSMSuThdRwRtStFrwdBkwdPos_Val_read>"
  ThdRwRtStPossV/1 -> Bus Selector1/1
  ThdRwRtStPoss/1 -> Bus Selector/1
  Bus Selector/2 -> [ThdRwRtStCshnFldUpwdDnwdPos]  "<IfVeSMSuThdRwRtStCshnFldUpwdDnwdPos_Val_read>"
  Bus Selector/1 -> [ThdRwRtStBkReclnUpwdDnwdPos]  "<IfVeSMSuThdRwRtStBkReclnUpwdDnwdPos_Val_read>"
  Bus Selector1/2 -> [ThdRwRtStCshnFldUpwdDnwdPosV]  "<IfVeSMSuThdRwRtStCshnFldUpwdDnwdPosV_Val_read>"
  Bus Selector1/3 -> [ThdRwRtStFrwdBkwdPosV]  "<IfVeSMSuThdRwRtStFrwdBkwdPosV_Val_read>"
  [R3Rt_CshnFldUpwdDnwd_TarPos] -> Bus Creator/2  "ThdRwRtStCshnFldUpwdDnwdTrgtPos"
  [R3RtReclnUpDn_TarPos] -> Bus Creator/1  "ThdRwRtStBkReclnUpwdDnwdTrgtPos"
  [R3Rt_FrwdBkwd_TarPos] -> Bus Creator/3  "ThdRwRtStFrwdBkwdTrgtPos"
  Bus Creator/1 -> R3Rt_TrgtPoss/1
  Bus Selector4/2 -> [CshnFldUpwdDnwdMovConfig]  "<CshnFldUpwdDnwdMovConfig>"
  Bus Selector4/1 -> [BkReclnUpwdDnwdMovConfig]  "<BkReclnUpwdDnwdMovConfig>"
  StConfig/1 -> Bus Selector4/1
  Bus Selector4/3 -> [FrwdBkwdMovConfig]  "<FrwdBkwdMovConfig>"
  [CshnFldUpwdDnwdMovConfig] -> R3Rt_CshnFldUpwdDnwd_Step1/14
  [FrwdBkwdMovConfig] -> R3RtReclnUpDn_Step2/14
  [BkReclnUpwdDnwdMovConfig] -> R3RtReclnUpDn_Step1/14
  [CntLow] -> R3RtReclnUpDn_Step1/15
  [CntLow] -> R3Rt_CshnFldUpwdDnwd_Step1/15
  PA_KeSMSuMdRetryTm1_Val/1 -> [CntLow]
  [CntLow] -> R3RtReclnUpDn_Step2/15
  [R3Rt_FrwdBkwd_TarPos] -> Relational Operator1/1
  Relational Operator1/1 -> Switch/2
  Constant1/1 -> Switch/3
  Constant/1 -> Switch/1
  Switch/1 -> R3Lt_SpdCtrl/1
  PA_KeSMSwDltTrgtPos_Val18/1 -> Relational Operator1/2
  ThdRwRtStFrwdCmdSrv/1 -> NOT/1
